simulink model "CW_Sim"  (R2024a)
settings: Solver=FixedStepAuto  StartTime=0.0  StopTime=2358720  FixedStep=120  RelTol=1e-3
values from neighbouring files (symbols this model uses):
  G = 6.674e-11    [CW_Driver.m]
  mE = 5.97219e24    (= 5.97219e+24)    [CW_Driver.m]
  mM = plot3(OM(mid,1)/1000,OM(mid,2)/1000,OM(mid,3)/1000,Marker="o",LineStyle="none",Color="red")    [CW_Driver.m]
  posE = [-xE 0 0]    [CW_Driver.m]
  posM = [xM 0 0]    [CW_Driver.m]
  posS = [xL2-(200*2000) 0 1000*2000]    [CW_Driver.m]
  velE = [0 -vE 0]    [CW_Driver.m]
  velM = [0 vM 0]    [CW_Driver.m]
  velS = [-0.00103491*2222.6 vSe+(0.004*2000) 0]    [CW_Driver.m]
settings Model: Creator=sgtjake2  LastModifiedBy=sgtjake2

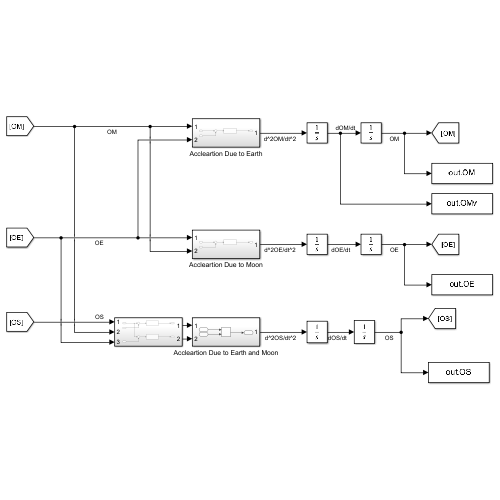
[thumbnail: Simulink's stored preview of the top-level diagram]
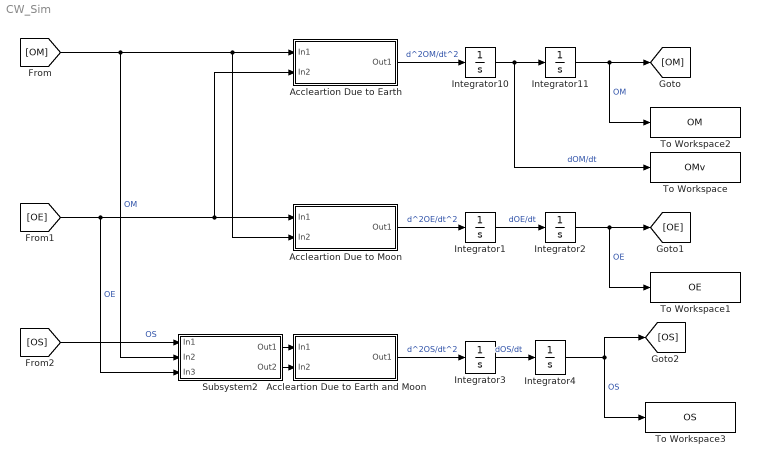
== system CW_Sim ==
  Accleartion Due to Earth : Subsystem
  Accleartion Due to Earth and Moon : Subsystem
  Accleartion Due to Moon : Subsystem
  Integrator1 : Integrator  InitialCondition=velE
  Integrator10 : Integrator  InitialCondition=velM
  Integrator11 : Integrator  InitialCondition=posM
  Integrator2 : Integrator  InitialCondition=posE
  Integrator3 : Integrator  InitialCondition=velS
  Integrator4 : Integrator  InitialCondition=posS
  Subsystem2 : Subsystem
  To Workspace : ToWorkspace  VariableName=OMv  SaveFormat=Timeseries  SampleTime=-1
  To Workspace1 : ToWorkspace  VariableName=OE  SaveFormat=Timeseries  SampleTime=-1
  To Workspace2 : ToWorkspace  VariableName=OM  SaveFormat=Timeseries  SampleTime=-1
  To Workspace3 : ToWorkspace  VariableName=OS  SaveFormat=Timeseries  SampleTime=-1
  wires:
  [OE] -> Subsystem2/3(In3), Accleartion Due to Moon/1(In1), Accleartion Due to Earth/2(In2)  "OE"
  [OM] -> Accleartion Due to Moon/2(In2), Accleartion Due to Earth/1(In1), Subsystem2/2(In2)  "OM"
  Integrator1/1 -> Integrator2/1  "dOE/dt"
  Accleartion Due to Moon/1(Out1) -> Integrator1/1  "d^2OE/dt^2"
  Integrator11/1 -> To Workspace2/1, [OM]  "OM"
  Accleartion Due to Earth/1(Out1) -> Integrator10/1  "d^2OM/dt^2"
  Integrator2/1 -> To Workspace1/1, [OE]  "OE"
  Integrator10/1 -> To Workspace/1, Integrator11/1  "dOM/dt"
  Integrator4/1 -> To Workspace3/1, [OS]  "OS"
  Accleartion Due to Earth and Moon/1(Out1) -> Integrator3/1  "d^2OS/dt^2"
  Subsystem2/2(Out2) -> Accleartion Due to Earth and Moon/2(In2)
  Subsystem2/1(Out1) -> Accleartion Due to Earth and Moon/1(In1)
  Integrator3/1 -> Integrator4/1  "dOS/dt"
  [OS] -> Subsystem2/1(In1)  "OS"

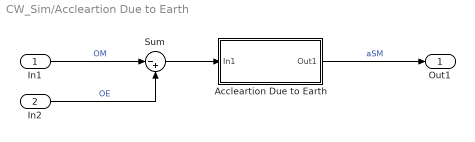
== system CW_Sim/Accleartion Due to Earth ==
  In1 : Inport
  In2 : Inport  Port=2
  Accleartion Due to Earth : Subsystem
  Sum : Sum  Inputs=|-+
  Out1 : Outport
  wires:
  Accleartion Due to Earth/1(Out1) -> Out1/1  "aSM"
  Sum/1 -> Accleartion Due to Earth/1(In1)
  In1/1 -> Sum/1  "OM"
  In2/1 -> Sum/2  "OE"

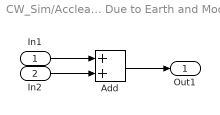
== system CW_Sim/Accleartion Due to Earth and Moon ==
  In1 : Inport
  In2 : Inport  Port=2
  Add : Sum
  Out1 : Outport
  wires:
  Add/1 -> Out1/1
  In1/1 -> Add/1
  In2/1 -> Add/2

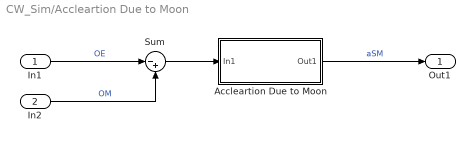
== system CW_Sim/Accleartion Due to Moon ==
  In1 : Inport
  In2 : Inport  Port=2
  Accleartion Due to Moon : Subsystem
  Sum : Sum  Inputs=|-+
  Out1 : Outport
  wires:
  Accleartion Due to Moon/1(Out1) -> Out1/1  "aSM"
  Sum/1 -> Accleartion Due to Moon/1(In1)
  In1/1 -> Sum/1  "OE"
  In2/1 -> Sum/2  "OM"

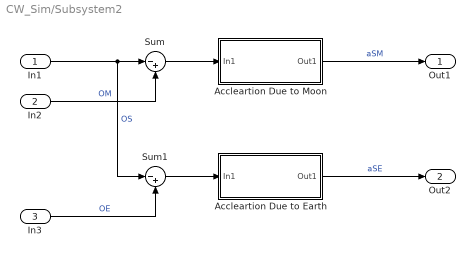
== system CW_Sim/Subsystem2 ==
  In1 : Inport
  In2 : Inport  Port=2
  In3 : Inport  Port=3
  Accleartion Due to Earth : Subsystem
  Accleartion Due to Moon : Subsystem
  Sum : Sum  Inputs=|-+
  Sum1 : Sum  Inputs=|-+
  Out1 : Outport
  Out2 : Outport  Port=2
  wires:
  Accleartion Due to Moon/1(Out1) -> Out1/1  "aSM"
  Sum/1 -> Accleartion Due to Moon/1(In1)
  In1/1 -> Sum1/1, Sum/1  "OS"
  In2/1 -> Sum/2  "OM"
  Sum1/1 -> Accleartion Due to Earth/1(In1)
  Accleartion Due to Earth/1(Out1) -> Out2/1  "aSE"
  In3/1 -> Sum1/2  "OE"

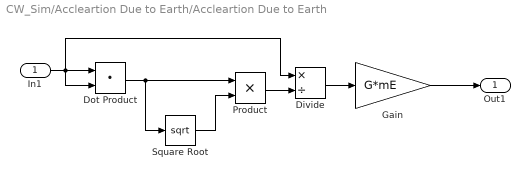
== system CW_Sim/Accleartion Due to Earth/Accleartion Due to Earth ==
  In1 : Inport
  Divide : Product  Inputs=*/
  Dot Product : DotProduct  OutDataTypeStr=Inherit: Inherit via internal rule
  Gain : Gain  Gain=G*mE
  Product : Product
  Square Root : Sqrt
  Out1 : Outport
  wires:
  In1/1 -> Divide/1, Dot Product/2, Dot Product/1
  Dot Product/1 -> Square Root/1, Product/1
  Square Root/1 -> Product/2
  Product/1 -> Divide/2
  Gain/1 -> Out1/1
  Divide/1 -> Gain/1

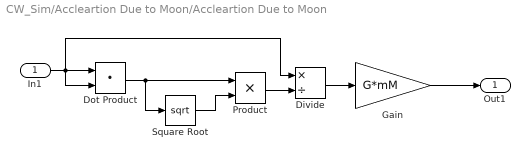
== system CW_Sim/Accleartion Due to Moon/Accleartion Due to Moon ==
  In1 : Inport
  Divide : Product  Inputs=*/
  Dot Product : DotProduct  OutDataTypeStr=Inherit: Inherit via internal rule
  Gain : Gain  Gain=G*mM
  Product : Product
  Square Root : Sqrt
  Out1 : Outport
  wires:
  In1/1 -> Divide/1, Dot Product/2, Dot Product/1
  Dot Product/1 -> Square Root/1, Product/1
  Square Root/1 -> Product/2
  Product/1 -> Divide/2
  Gain/1 -> Out1/1
  Divide/1 -> Gain/1

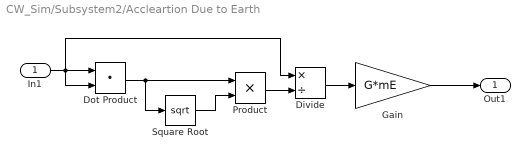
== system CW_Sim/Subsystem2/Accleartion Due to Earth ==
  In1 : Inport
  Divide : Product  Inputs=*/
  Dot Product : DotProduct  OutDataTypeStr=Inherit: Inherit via internal rule
  Gain : Gain  Gain=G*mE
  Product : Product
  Square Root : Sqrt
  Out1 : Outport
  wires:
  In1/1 -> Divide/1, Dot Product/2, Dot Product/1
  Dot Product/1 -> Square Root/1, Product/1
  Square Root/1 -> Product/2
  Product/1 -> Divide/2
  Gain/1 -> Out1/1
  Divide/1 -> Gain/1

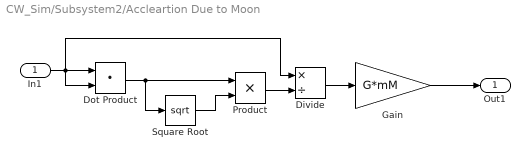
== system CW_Sim/Subsystem2/Accleartion Due to Moon ==
  In1 : Inport
  Divide : Product  Inputs=*/
  Dot Product : DotProduct  OutDataTypeStr=Inherit: Inherit via internal rule
  Gain : Gain  Gain=G*mM
  Product : Product
  Square Root : Sqrt
  Out1 : Outport
  wires:
  In1/1 -> Divide/1, Dot Product/2, Dot Product/1
  Dot Product/1 -> Square Root/1, Product/1
  Square Root/1 -> Product/2
  Product/1 -> Divide/2
  Gain/1 -> Out1/1
  Divide/1 -> Gain/1
